simulink model "Simulink_Timing_Legend"  (R2025b)
settings: Solver=VariableStepAuto  StartTime=0.0  StopTime=10.0  RelTol=1e-3
settings Model: Creator=georg  LastModifiedBy=georg

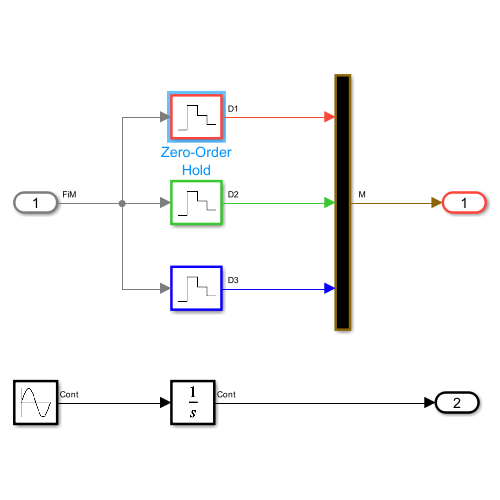
[thumbnail: Simulink's stored preview of the top-level diagram]
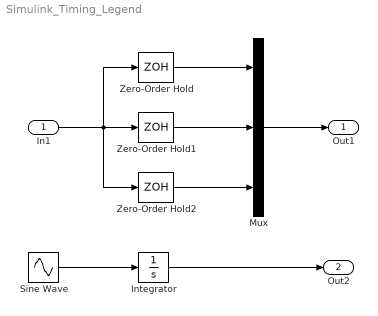
== system Simulink_Timing_Legend ==
  In1 : Inport  SampleTime=[0,1]
  Integrator : Integrator
  Mux : Mux  Inputs=3
  Sine Wave : Sin  SampleTime=0
  Zero-Order Hold : ZeroOrderHold  SampleTime=[1,0]
  Zero-Order Hold1 : ZeroOrderHold  SampleTime=2
  Zero-Order Hold2 : ZeroOrderHold  SampleTime=3
  Out1 : Outport
  Out2 : Outport  Port=2
  wires:
  In1/1 -> Zero-Order Hold1/1, Zero-Order Hold/1, Zero-Order Hold2/1
  Zero-Order Hold/1 -> Mux/1
  Zero-Order Hold1/1 -> Mux/2
  Zero-Order Hold2/1 -> Mux/3
  Mux/1 -> Out1/1
  Sine Wave/1 -> Integrator/1
  Integrator/1 -> Out2/1
